simulink model "Fuzzy_ROS_ROSPath"  (R2019a)
settings: Solver=FixedStepAuto  StartTime=0.0  StopTime=1000.0  FixedStep=0.01  RelTol=1e-3
values from neighbouring files (symbols this model uses):
  path = [      0         0 ... (first row only)    [JACKAL_dynamic_model.m]    (also in Jackal_kinematic_model.m = [0 0;path]; RLLOOP2.m = [5,   0)
  speed = 1.5    [JACKAL_dynamic_model.m]    (also in Jackal_kinematic_model.m = 2)
undefined symbols (not defined in the file or in its folder): Angular, Linear
libraries: robotlib x4, fuzblock x1, simulink x1
settings Model: Creator=dev  LastModifiedBy=12248

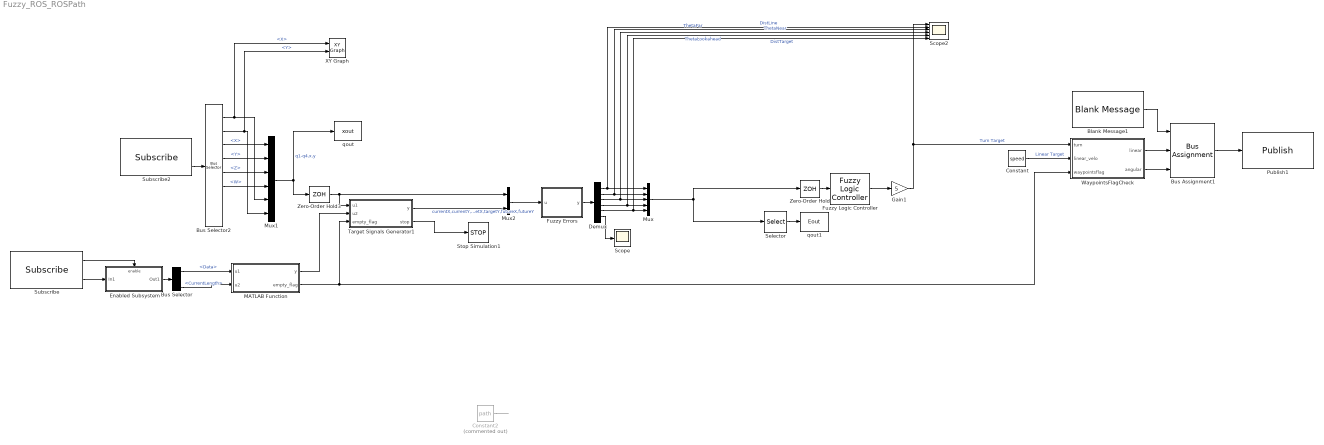
== system Fuzzy_ROS_ROSPath ==
  Blank Message1 : robotlib/Blank Message  messageClass=Message  entityType=geometry_msgs/Twist  messageType=geometry_msgs/Twist  SampleTime=inf
      settings: SourceProductBaseCode=RO
  Bus Assignment1 : BusAssignment  AssignedSignals=Linear.X,Angular.Z
  Bus Selector : BusSelector  OutputSignals=Data,Data_SL_Info.ReceivedLength,Data_SL_Info.CurrentLength
  Bus Selector2 : BusSelector  OutputSignals=Pose.Pose.Position.X,Pose.Pose.Position.Y,Pose.Pose.Orientation.X,Pose.Pose.Orientation.Y,Pose.Pose.Orientation.Z,Pose.Pose.Orientation.W,Twist.Twist.Linear.X,Twist.Twist.Angular.Z
  Constant : Constant  Value=speed
  Constant2 : Constant  Commented=on  Value=path
  Demux : Demux  Outputs=6
  Enabled Subsystem : Subsystem  TreatAsAtomicUnit=on
  Fuzzy Errors : MATLAB Function  TreatAsAtomicUnit=on
  Fuzzy Logic Controller : fuzblock/Fuzzy Logic  Controller  FIS='fuzzyControlDistSlow.fis'  OutputSampleNumber=3000  DataType=double  FuzzifiedInputs=off  RuleFiringStrengths=on  RuleOutputs=off  AggregatedOutputs=on  SimulateUsing=Code generation  OutOfRangeInputValueMessage=warning  NoRuleFiredMessage=warning  EmptyOutputFuzzySetMessage=warning
  Gain1 : Gain  Gain=5
  MATLAB Function : MATLAB Function  TreatAsAtomicUnit=on
  Mux : Mux  Inputs=5
  Mux1 : Mux  Inputs=6
  Mux2 : Mux  Inputs=2
  Publish1 : robotlib/Publish  topicSource=Select from ROS network  topic=/cmd_vel  messageType=geometry_msgs/Twist  messageQueueLength=1
      settings: SourceProductBaseCode=RO
  Scope : Scope
  Scope2 : Scope  NumInputPorts=6
  Selector : Selector  InputPortWidth=5  IndexOptions=Index vector (dialog)  Indices=[1]  OutputSizes=1
  Stop Simulation1 : Stop
  Subscribe : robotlib/Subscribe  topicSource=Select from ROS network  topic=/path_publisher  messageType=std_msgs/Float32MultiArray  sampleTime=-1  messageQueueLength=1
      settings: SourceProductBaseCode=RO
  Subscribe2 : robotlib/Subscribe  topicSource=Select from ROS network  topic=/odometry/filtered  messageType=nav_msgs/Odometry  sampleTime=-1  messageQueueLength=1
      settings: SourceProductBaseCode=RO
  Target Signals Generator1 : MATLAB Function  TreatAsAtomicUnit=on
  WaypointsFlagCheck : MATLAB Function  TreatAsAtomicUnit=on
  XY Graph : simulink/Sinks/XY Graph  xmin=-5  xmax=5  ymin=-5  ymax=5  st=-1
  Zero-Order Hold : ZeroOrderHold  SampleTime=.001
  Zero-Order Hold3 : ZeroOrderHold  SampleTime=.001
  qout : ToWorkspace  VariableName=xout  SampleTime=-1
  qout1 : ToWorkspace  VariableName=Eout  SampleTime=-1
  wires:
  Constant/1 -> WaypointsFlagCheck/2(linear_velo)  "Linear Target"
  Bus Assignment1/1 -> Publish1/1
  Blank Message1/1 -> Bus Assignment1/1
  Bus Selector2/2 -> Mux1/6, XY Graph/2  "<Y>"
  Bus Selector2/3 -> Mux1/1  "<X>"
  Bus Selector2/4 -> Mux1/2  "<Y>"
  Bus Selector2/6 -> Mux1/4  "<W>"
  Mux1/1 -> Zero-Order Hold3/1, qout/1  "q1-q4,x,y"
  Bus Selector2/1 -> Mux1/5, XY Graph/1  "<X>"
  Bus Selector2/5 -> Mux1/3  "<Z>"
  Subscribe2/2 -> Bus Selector2/1
  Demux/6 -> Scope/1
  Demux/3 -> Scope2/4, Mux/3  "ThetaNear"
  Fuzzy Logic Controller/1 -> Gain1/1
  Mux/1 -> Selector/1, Zero-Order Hold/1
  Demux/5 -> Scope2/6, Mux/5  "DistTarget"
  Demux/1 -> Scope2/2, Mux/1  "DistLine"
  Demux/4 -> Scope2/5, Mux/4  "ThetaLookahead"
  Demux/2 -> Scope2/3, Mux/2  "ThetaFar"
  Target Signals Generator1/2(stop) -> Stop Simulation1/1
  Fuzzy Errors/1(y) -> Demux/1
  Target Signals Generator1/1(y) -> Mux2/2  "currentX,currentY,targetX,targetY,futureX,futureY"
  Zero-Order Hold/1 -> Fuzzy Logic Controller/1
  Zero-Order Hold3/1 -> Target Signals Generator1/1(u1), Mux2/1
  Selector/1 -> qout1/1
  Gain1/1 -> WaypointsFlagCheck/1(turn), Scope2/1  "Turn Target"
  Mux2/1 -> Fuzzy Errors/1(u)
  Subscribe/2 -> Enabled Subsystem/1(In1)
  Enabled Subsystem/1(Out1) -> Bus Selector/1
  Bus Selector/3 -> MATLAB Function/2(u2)  "<CurrentLength>"
  Subscribe/1 -> Enabled Subsystem/Enable
  Bus Selector/1 -> MATLAB Function/1(u1)  "<Data>"
  Constant2/1 -> ?
  MATLAB Function/2(empty_flag) -> Target Signals Generator1/3(empty_flag), WaypointsFlagCheck/3(waypointsflag)
  WaypointsFlagCheck/1(linear) -> Bus Assignment1/2
  WaypointsFlagCheck/2(angular) -> Bus Assignment1/3
  MATLAB Function/1(y) -> Target Signals Generator1/2(u2)

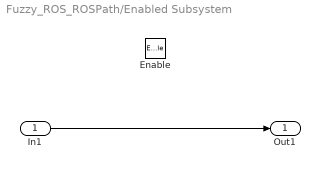
== system Fuzzy_ROS_ROSPath/Enabled Subsystem ==
  In1 : Inport
  Enable : EnablePort
  Out1 : Outport
  wires:
  In1/1 -> Out1/1

== matlab function Fuzzy_ROS_ROSPath/WaypointsFlagCheck ==
  data: turn input; linear output; linear_velo input; waypointsflag input; angular output
function [linear, angular] = fcn(turn, linear_velo, waypointsflag)

if(waypointsflag==0)
    linear=0;
    angular=0;
end

if(waypointsflag==1)
    linear=linear_velo;
    angular=turn;
end

== matlab function Fuzzy_ROS_ROSPath/MATLAB Function ==
  data: u1 input; y output size=256; u2 input; empty_flag output
function [y, empty_flag] = fcn(u1,u2)
u1 = double(u1);
test_array = u1(1:6);
empty_flag = 0;
path_length = u2;
disp(path_length)
path = [0, 0;100, 100];

for i = 1:6 
    if test_array(i) ~= 0
        empty_flag = 1;
        break
    end
end

if empty_flag == 0
    for i = 1 : pathlength/2
        path(i,:) = [u1(2*i-1),u1(2i)];
    end
end
y = path;

== matlab function Fuzzy_ROS_ROSPath/Fuzzy Errors ==
  settings: updateMethod=DISCRETE
  data: u input; y output
function y  = fcn(u)

%jackal dyanamic model
pos=[u(5) u(6)]; % [x,y]
q=[u(1) u(2) u(3) u(4)]; % orientation quaternion
currentAngle=atan2(2*(q(1)*q(4)+q(2)*q(3)),1-2*(q(3)^2+q(4)^2));% Angle robot is currently facing

currentPoint=[u(7) u(8)];
target=[u(9) u(10)];
future=[u(11) u(12)];

A = [(currentPoint(2)-target(2)), target(1)-currentPoint(1); target(1)-currentPoint(1), target(2)-currentPoint(2)];
b = [ target(1)*currentPoint(2)-currentPoint(1)*target(2); pos(1)*(target(1)-currentPoint(1)) + pos(2)*(target(2)-currentPoint(2))];
proj = (A\b)'; %projected point on the line between  .

d = ( pos(1)-currentPoint(1) )*(target(2)-currentPoint(2)) - (pos(2)-currentPoint(2))*(target(1)-currentPoint(1));

if ( d >0)
    side = 1;
elseif ( d < 0)
    side = -1;
else
    side = 0;
end

distanceLine=norm(pos-proj)*side;
distanceTarget=sqrt((target(1)-pos(1))^2+(target(2)-pos(2))^2);

% %wrap to +/-pi
% if((currentAngle < -pi) || (pi < currentAngle))
%     currentAngle = mod(currentAngle+pi, 2*pi)-pi;
% end

farTarget=[.95*proj(1)+.05*target(1) .95*proj(2)+.05*target(2)];

th1 = atan2(farTarget(2)-pos(2), farTarget(1)-pos(1));
th2 = atan2(target(2)-currentPoint(2), target(1)-currentPoint(1));
th3 = atan2(future(2)-target(2), future(1)-target(1)); 

ThetaFar=th1-currentAngle;
ThetaNear=th2-currentAngle;
ThetaLookahead=th3-currentAngle;

%wrap to +/-pi
if((ThetaFar < -pi) || (pi < ThetaFar))
    ThetaFar = mod(ThetaFar+pi, 2*pi)-pi;
end

%wrap to +/-pi
if((ThetaNear < -pi) || (pi < ThetaNear))
    ThetaNear = mod(ThetaNear+pi, 2*pi)-pi;
end

%wrap to +/-pi
if((ThetaLookahead < -pi) || (pi < ThetaLookahead))
    ThetaLookahead = mod(ThetaLookahead+pi, 2*pi)-pi;
end

y = [distanceLine;ThetaFar;ThetaNear;ThetaLookahead;distanceTarget;currentAngle];

== matlab function Fuzzy_ROS_ROSPath/Target Signals Generator1 ==
  data: u1 input; y output; u2 input; stop output; empty_flag input
function [y,stop] = fcn(u1,u2,empty_flag)

persistent pathcount;
persistent pathlength;
persistent path; %error in code, initially used path but this is already a matlab function
persistent pathPre;
persistent waypointsflag;
persistent insideflag;

if isempty(waypointsflag)
    waypointsflag=0;
    insideflag=0;
end

if (isempty(pathcount)||waypointsflag==0) %until the first time we get a real path, keep setting the fake paths as path to do control on
    if (insideflag==0)
        pathcount=1;     
        pathPre=u2;
        [pathlength,~]=size(pathPre);  
        path=[pathPre; pathPre(pathlength,1)+100 pathPre(pathlength,2)+100]; %sim takes multiple iterations to stop after reaching final point, so this prevents it from breaking
        insideflag=1; %we went in here once so dont go in here ever again
    end
end

waypointsflag=empty_flag;

pos=[u1(5) u1(6)]; % [x,y] 
currentPoint=path(pathcount,:);
target=path(pathcount+1,:);

A = [(currentPoint(2)-target(2)), target(1)-currentPoint(1); target(1)-currentPoint(1), target(2)-currentPoint(2)];
b = [ target(1)*currentPoint(2)-currentPoint(1)*target(2); pos(1)*(target(1)-currentPoint(1)) + pos(2)*(target(2)-currentPoint(2))];
proj = (A\b)'; %projected point on the line between  .
projLen=dot(proj-currentPoint,target-currentPoint)/norm(target-currentPoint)^2; %the distance along the projected line, where 0 is the start point and 1 is the end point

distErr=sqrt((target(2)-pos(2))^2+(target(1)-pos(1))^2);

if ((projLen>1)||(distErr<.175))
    pathcount=pathcount+1;
end

%check if at destination and terminate sim if there
pathflag=0;
if (pathcount==pathlength)
    
    pathflag=1;
end

if ((pathcount==(pathlength-1))||(pathcount==(pathlength)))
    a=path(pathcount,:);
    b=path(pathcount+1,:);
    post=path(pathcount+1,:);
else
    a=path(pathcount,:);
    b=path(pathcount+1,:);
    post=path(pathcount+2,:);
end

y = [a(1);a(2);b(1);b(2);post(1);post(2)];
stop=pathflag;
